simulink library "tangVecToPath"  (R2018b)
settings: Solver=VariableStepAuto  StartTime=0.0  StopTime=10.0  RelTol=1e-3
libraries: dspmathops x4
settings Model: Creator=James Reed  LastModifiedBy=James Reed

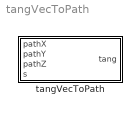
== system tangVecToPath ==
  tangVecToPath : Subsystem

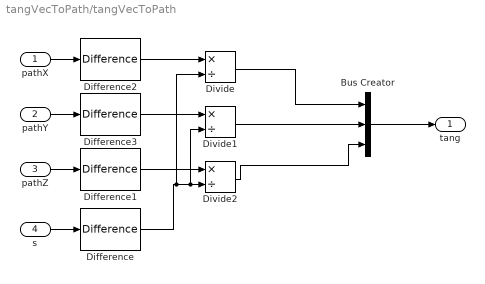
== system tangVecToPath/tangVecToPath ==
  "pathX " : Inport
  pathY : Inport  Port=2
  pathZ : Inport  Port=3
  "s " : Inport  Port=4
  Bus Creator : BusCreator  Inputs=3
  Difference{,1..3} (4 alike) : dspmathops/Difference  Run=No  dim=Columns  Dimension=1  roundingMode=Floor  overflowMode=off  outputDataTypeStr=Inherit: Same as accumulator  outputMin=[]  outputMax=[]  outputLastDataTypeStr=Inherit: Same as accumulator
      settings: SourceProductName=DSP System Toolbox  SourceProductBaseCode=DS
  Divide : Product  Inputs=*/
  Divide1 : Product  Inputs=*/
  Divide2 : Product  Inputs=*/
  tang : Outport
  wires:
  Divide2/1 -> Bus Creator/3
  Divide/1 -> Bus Creator/1
  Bus Creator/1 -> tang/1
  pathZ/1 -> Difference1/1
  "s "/1 -> Difference/1
  pathY/1 -> Difference3/1
  Difference3/1 -> Divide1/1
  Divide1/1 -> Bus Creator/2
  Difference2/1 -> Divide/1
  Difference1/1 -> Divide2/1
  Difference/1 -> Divide/2, Divide1/2, Divide2/2
  "pathX "/1 -> Difference2/1
